simulink model "sampleModel2047"  (R2023a)
settings: Solver=VariableStepAuto  StartTime=0.0  StopTime=10.0  RelTol=1e-3
libraries: hdlsllib x5, simulink x1
settings Model: Creator=user1  LastModifiedBy=user1

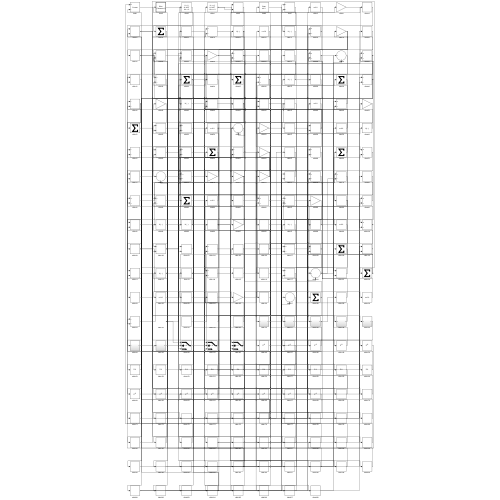
[thumbnail: Simulink's stored preview of the top-level diagram]
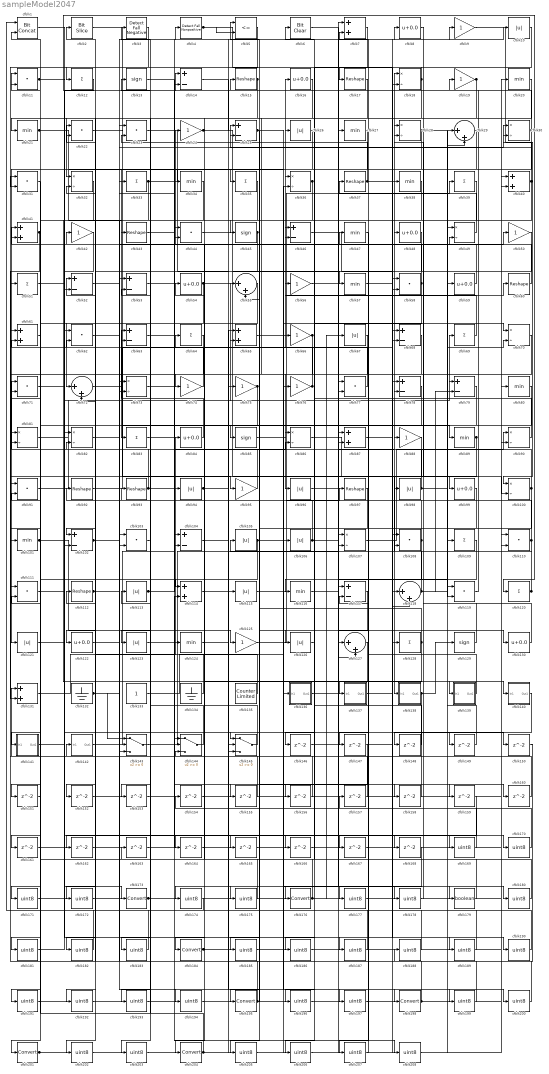
== system sampleModel2047 ==
  cfblk1 : hdlsllib/Logic and Bit Operations/Bit Concat  numInputs=2
  cfblk{10,26,67,94,96,98,105..106,113,115,121,123,126} (13 alike) : Abs  SaturateOnIntegerOverflow=off
  cfblk{18,28,30,32,36,49,70,73,81..82,86,90,100,107} (14 alike) : Product  Inputs=*/  RndMeth=Zero  SaturateOnIntegerOverflow=on
  cfblk{20..21,27,34,38,47,57,80,89,101,116,124} (12 alike) : MinMax
  cfblk{14,25,46,52..53,63,68,78..79,102,104,117} (12 alike) : Sum  Inputs=+-
  cfblk{11,22..23,31,44,58,62,71,77,91,103,108,110..111,119} (15 alike) : DotProduct  OutDataTypeStr=Inherit: Inherit via internal rule
  cfblk{12,33,35,39,51,64,69,83,109,120,128} (11 alike) : Sum  Inputs=+
  cfblk{15,17,37,43,60,92..93,97,112} (9 alike) : Reshape
  cfblk{7,40..41,61,65,87,114,131} (8 alike) : Sum
  cfblk{29,55,72,118,127} (5 alike) : Sum  Inputs=|++
  cfblk{8,16,48,54,59,84,99,122,130} (9 alike) : Bias  Bias=0.0  SaturateOnIntegerOverflow=off
  cfblk{9,19,24,42,50,56,66,74..76,88,95,125} (13 alike) : Gain
  cfblk{13,45,85,129} (4 alike) : Signum
  cfblk132 : Ground
  cfblk133 : Constant  SampleTime=-1
  cfblk134 : Ground
  cfblk135 : hdlsllib/Sources/Counter Limited  uplimit=7  tsamp=-1
  cfblk136 : Subsystem
      settings: LibrarySourceBlock=|
      | hdlsllib/Ports &
      | Subsystems/Subsystem
  cfblk137 : Subsystem
      settings: LibrarySourceBlock=|
      | hdlsllib/Ports &
      | Subsystems/Subsystem
  cfblk138 : Subsystem
      settings: LibrarySourceBlock=|
      | hdlsllib/Ports &
      | Subsystems/Subsystem
  cfblk139 : Subsystem
      settings: LibrarySourceBlock=|
      | hdlsllib/Ports &
      | Subsystems/Subsystem
  cfblk140 : Subsystem
      settings: LibrarySourceBlock=|
      | hdlsllib/Ports &
      | Subsystems/Subsystem
  cfblk141 : Subsystem
      settings: LibrarySourceBlock=|
      | hdlsllib/Ports &
      | Subsystems/Subsystem
  cfblk142 : Subsystem
      settings: LibrarySourceBlock=|
      | hdlsllib/Ports &
      | Subsystems/Subsystem
  cfblk143 : Switch  SaturateOnIntegerOverflow=off  InputSameDT=off
  cfblk144 : Switch  SaturateOnIntegerOverflow=off  InputSameDT=off
  cfblk145 : Switch  SaturateOnIntegerOverflow=off  InputSameDT=off
  cfblk{146..168} (23 alike) : Delay  SampleTime=1
  cfblk{169..172,174..175,177..178,180..183,185..194,196..197,199..200,202..203,205..208} (32 alike) : DataTypeConversion  OutDataTypeStr=uint8  SaturateOnIntegerOverflow=off  RndMeth=Floor
  cfblk{173,176,184,195,198,201,204} (7 alike) : DataTypeConversion  SaturateOnIntegerOverflow=off  RndMeth=Floor
  cfblk179 : DataTypeConversion  OutDataTypeStr=boolean  SaturateOnIntegerOverflow=off  RndMeth=Floor
  cfblk2 : hdlsllib/Logic and Bit Operations/Bit Slice  lidx=7  ridx=0
  cfblk3 : hdlsllib/Logic and Bit Operations/Detect Fall Negative  vinit=0  OutDataTypeStr=boolean
  cfblk4 : hdlsllib/Logic and Bit Operations/Detect Fall Nonpositive  vinit=0  OutDataTypeStr=boolean
  cfblk5 : RelationalOperator  Operator=<=  OutDataTypeStr=boolean  InputSameDT=off
  cfblk6 : simulink/Logic and Bit Operations/Bit Clear  iBit=0
      settings: LibrarySourceBlock=|
      | hdlsllib/Logic and Bit
      | Operations/Bit Clear
  wires:
  cfblk40/1 -> cfblk102/2, cfblk30/1, cfblk25/2, cfblk162/1, cfblk193/1
  cfblk3/1 -> cfblk12/1
  cfblk55/1 -> cfblk72/1
  cfblk92/1 -> cfblk15/1
  cfblk9/1 -> cfblk100/1
  cfblk19/1 -> cfblk74/1, cfblk102/1, cfblk145/3
  cfblk44/1 -> cfblk57/1
  cfblk32/1 -> cfblk137/1(In1)
  cfblk130/1 -> cfblk42/1
  cfblk26/1 -> cfblk121/1
  cfblk107/1 -> cfblk90/1
  cfblk106/1 -> cfblk64/1, cfblk150/1
  cfblk85/1 -> cfblk60/1
  cfblk2/1 -> cfblk89/1
  cfblk28/1 -> cfblk100/2, cfblk183/1
  cfblk110/1 -> cfblk84/1, cfblk108/2
  cfblk86/1 -> cfblk99/1
  cfblk142/1(Out1) -> cfblk94/1
  cfblk102/1 -> cfblk4/1, cfblk30/2
  cfblk125/1 -> cfblk39/1
  cfblk12/1 -> cfblk120/1
  cfblk22/1 -> cfblk95/1
  cfblk115/1 -> cfblk97/1
  cfblk134/1 -> cfblk104/1
  cfblk66/1 -> cfblk96/1, cfblk185/1
  cfblk69/1 -> cfblk16/1
  cfblk54/1 -> cfblk138/1(In1), cfblk141/1(In1)
  cfblk80/1 -> cfblk103/2
  cfblk21/1 -> cfblk83/1, cfblk136/1(In1)
  cfblk144/1 -> cfblk93/1
  cfblk131/1 -> cfblk104/2
  cfblk70/1 -> cfblk86/1
  cfblk53/1 -> cfblk198/1
  cfblk108/1 -> cfblk2/1, cfblk206/1
  cfblk118/1 -> cfblk18/1, cfblk79/2, cfblk70/2
  cfblk91/1 -> cfblk69/1
  cfblk74/1 -> cfblk52/1
  cfblk95/1 -> cfblk71/1
  cfblk77/1 -> cfblk36/1
  cfblk143/1 -> cfblk27/1
  cfblk11/1 -> cfblk145/1, cfblk170/1
  cfblk24/1 -> cfblk119/1, cfblk8/1
  cfblk27/1 -> cfblk43/1
  cfblk39/1 -> cfblk45/1
  cfblk136/1(Out1) -> cfblk88/1
  cfblk129/1 -> cfblk28/1
  cfblk138/1(Out1) -> cfblk131/1, cfblk129/1
  cfblk81/1 -> cfblk55/1
  cfblk145/1 -> cfblk54/1
  cfblk120/1 -> cfblk19/1, cfblk5/1
  cfblk46/1 -> cfblk118/1
  cfblk18/1 -> cfblk17/1, cfblk146/1
  cfblk117/1 -> cfblk195/1
  cfblk105/1 -> cfblk106/1, cfblk151/1
  cfblk1/1 -> cfblk173/1
  cfblk50/1 -> cfblk114/1
  cfblk84/1 -> cfblk63/1
  cfblk119/1 -> cfblk49/2
  cfblk90/1 -> cfblk26/1
  cfblk16/1 -> cfblk32/1
  cfblk15/1 -> cfblk21/1, cfblk144/2
  cfblk48/1 -> cfblk123/1
  cfblk45/1 -> cfblk122/1, cfblk73/2
  cfblk99/1 -> cfblk116/1
  cfblk25/1 -> cfblk55/2, cfblk70/1
  cfblk75/1 -> cfblk85/1, cfblk143/3
  cfblk71/1 -> cfblk82/1
  cfblk8/1 -> cfblk98/1
  cfblk62/1 -> cfblk47/1
  cfblk72/1 -> cfblk58/1
  cfblk59/1 -> cfblk28/2
  cfblk76/1 -> cfblk11/1, cfblk63/2
  cfblk121/1 -> cfblk139/1(In1)
  cfblk49/1 -> cfblk37/1
  cfblk10/1 -> cfblk58/2
  cfblk63/1 -> cfblk140/1(In1)
  cfblk64/1 -> cfblk131/2
  cfblk139/1(Out1) -> cfblk41/1
  cfblk5/1 -> cfblk31/2
  cfblk122/1 -> cfblk73/1
  cfblk41/1 -> cfblk81/2, cfblk51/1
  cfblk89/1 -> cfblk107/2, cfblk82/2
  cfblk116/1 -> cfblk50/1
  cfblk112/1 -> cfblk34/1, cfblk152/1
  cfblk96/1 -> cfblk130/1
  cfblk113/1 -> cfblk46/1, cfblk10/1
  cfblk100/1 -> cfblk48/1, cfblk156/1
  cfblk94/1 -> cfblk160/1, cfblk200/1
  cfblk114/1 -> cfblk115/1
  cfblk37/1 -> cfblk3/1, cfblk9/1
  cfblk93/1 -> cfblk62/2, cfblk65/2
  cfblk88/1 -> cfblk111/1
  cfblk83/1 -> cfblk86/2
  cfblk128/1 -> cfblk25/1, cfblk164/1
  cfblk135/1 -> cfblk92/1
  cfblk133/1 -> cfblk36/2
  cfblk58/1 -> cfblk126/1, cfblk44/1, cfblk22/2
  cfblk79/1 -> cfblk101/1
  cfblk132/1 -> cfblk33/1, cfblk143/1, cfblk22/1
  cfblk4/1 -> cfblk128/1, cfblk5/2
  cfblk36/1 -> cfblk91/1, cfblk143/2
  cfblk78/1 -> cfblk176/1
  cfblk33/1 -> cfblk35/1, cfblk191/1
  cfblk103/1 -> cfblk23/2
  cfblk23/1 -> cfblk75/1
  cfblk13/1 -> cfblk144/1
  cfblk127/1 -> cfblk204/1
  cfblk60/1 -> cfblk24/1
  cfblk20/1 -> cfblk184/1
  cfblk56/1 -> cfblk119/2
  cfblk30/1 -> cfblk14/2, cfblk165/1, cfblk166/1
  cfblk42/1 -> cfblk52/2
  cfblk98/1 -> cfblk59/1, cfblk56/1
  cfblk101/1 -> cfblk125/1, cfblk14/1
  cfblk141/1(Out1) -> cfblk79/1
  cfblk68/1 -> cfblk201/1
  cfblk146/1 -> cfblk118/2
  cfblk47/1 -> cfblk147/1
  cfblk140/1(Out1) -> cfblk148/1
  cfblk148/1 -> cfblk46/2
  cfblk104/1 -> cfblk149/1
  cfblk149/1 -> cfblk49/1
  cfblk151/1 -> cfblk41/2
  cfblk152/1 -> cfblk65/1
  cfblk34/1 -> cfblk153/1
  cfblk153/1 -> cfblk107/1
  cfblk154/1 -> cfblk110/2
  cfblk123/1 -> cfblk155/1
  cfblk155/1 -> cfblk23/1
  cfblk156/1 -> cfblk91/2
  cfblk157/1 -> cfblk103/1
  cfblk14/1 -> cfblk158/1
  cfblk158/1 -> cfblk81/1
  cfblk57/1 -> cfblk159/1
  cfblk160/1 -> cfblk77/1
  cfblk31/1 -> cfblk161/1
  cfblk161/1 -> cfblk90/2
  cfblk162/1 -> cfblk32/2
  cfblk163/1 -> cfblk114/2
  cfblk164/1 -> cfblk144/3
  cfblk111/1 -> cfblk167/1
  cfblk167/1 -> cfblk18/2
  cfblk43/1 -> cfblk168/1
  cfblk124/1 -> cfblk169/1
  cfblk169/1 -> cfblk154/1
  cfblk170/1 -> cfblk124/1
  cfblk38/1 -> cfblk171/1
  cfblk171/1 -> cfblk110/1
  cfblk67/1 -> cfblk172/1
  cfblk172/1 -> cfblk38/1
  cfblk173/1 -> cfblk40/2, cfblk113/1
  cfblk168/1 -> cfblk174/1
  cfblk174/1 -> cfblk1/1
  cfblk147/1 -> cfblk175/1
  cfblk175/1 -> cfblk1/2
  cfblk176/1 -> cfblk111/2, cfblk44/2, cfblk72/2, cfblk67/1
  cfblk65/1 -> cfblk177/1
  cfblk177/1 -> cfblk78/1
  cfblk166/1 -> cfblk178/1
  cfblk178/1 -> cfblk78/2
  cfblk137/1(Out1) -> cfblk179/1
  cfblk179/1 -> cfblk6/1
  cfblk6/1 -> cfblk180/1
  cfblk180/1 -> cfblk13/1
  cfblk61/1 -> cfblk181/1
  cfblk181/1 -> cfblk62/1
  cfblk35/1 -> cfblk182/1
  cfblk182/1 -> cfblk61/1
  cfblk183/1 -> cfblk61/2
  cfblk184/1 -> cfblk108/1, cfblk197/1
  cfblk185/1 -> cfblk20/1
  cfblk7/1 -> cfblk186/1
  cfblk186/1 -> cfblk77/2
  cfblk52/1 -> cfblk187/1
  cfblk187/1 -> cfblk7/1
  cfblk150/1 -> cfblk188/1
  cfblk188/1 -> cfblk7/2
  cfblk87/1 -> cfblk189/1
  cfblk189/1 -> cfblk142/1(In1)
  cfblk51/1 -> cfblk190/1
  cfblk190/1 -> cfblk87/1
  cfblk191/1 -> cfblk87/2
  cfblk29/1 -> cfblk192/1
  cfblk192/1 -> cfblk76/1
  cfblk193/1 -> cfblk29/1
  cfblk82/1 -> cfblk194/1
  cfblk194/1 -> cfblk29/2
  cfblk195/1 -> cfblk11/2, cfblk112/1, cfblk105/1
  cfblk126/1 -> cfblk196/1
  cfblk196/1 -> cfblk117/1
  cfblk197/1 -> cfblk117/2
  cfblk198/1 -> cfblk40/1, cfblk31/1
  cfblk165/1 -> cfblk199/1
  cfblk199/1 -> cfblk53/1
  cfblk200/1 -> cfblk53/2
  cfblk201/1 -> cfblk66/1, cfblk145/2, cfblk80/1
  cfblk159/1 -> cfblk202/1
  cfblk202/1 -> cfblk68/1
  cfblk17/1 -> cfblk203/1
  cfblk203/1 -> cfblk68/2
  cfblk204/1 -> cfblk163/1, cfblk71/2
  cfblk97/1 -> cfblk205/1
  cfblk205/1 -> cfblk127/1
  cfblk206/1 -> cfblk127/2
  cfblk109/1 -> cfblk207/1
  cfblk207/1 -> cfblk157/1
  cfblk73/1 -> cfblk208/1
  cfblk208/1 -> cfblk109/1

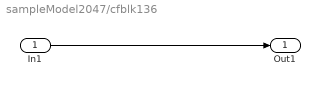
== system sampleModel2047/cfblk136 ==
  In1 : Inport
  Out1 : Outport
  wires:
  In1/1 -> Out1/1

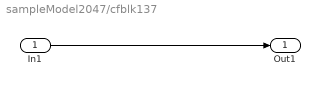
== system sampleModel2047/cfblk137 ==
  In1 : Inport
  Out1 : Outport
  wires:
  In1/1 -> Out1/1

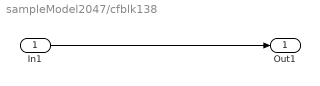
== system sampleModel2047/cfblk138 ==
  In1 : Inport
  Out1 : Outport
  wires:
  In1/1 -> Out1/1

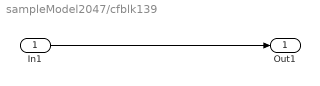
== system sampleModel2047/cfblk139 ==
  In1 : Inport
  Out1 : Outport
  wires:
  In1/1 -> Out1/1

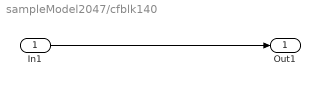
== system sampleModel2047/cfblk140 ==
  In1 : Inport
  Out1 : Outport
  wires:
  In1/1 -> Out1/1

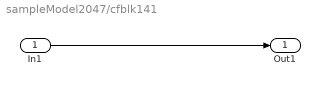
== system sampleModel2047/cfblk141 ==
  In1 : Inport
  Out1 : Outport
  wires:
  In1/1 -> Out1/1

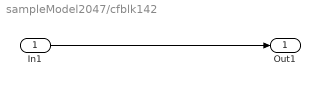
== system sampleModel2047/cfblk142 ==
  In1 : Inport
  Out1 : Outport
  wires:
  In1/1 -> Out1/1
